simulink model "castor"  (R2021b)
settings: Solver=VariableStepAuto  StartTime=0.0  StopTime=10  MaxStep=0.01  RelTol=1e-3
settings Model: Creator=Daniel  LastModifiedBy=Daniel

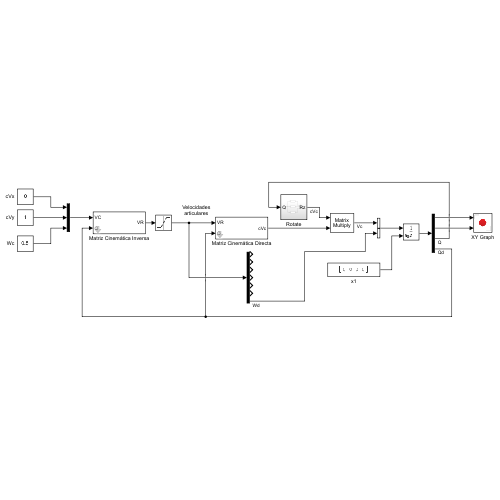
[thumbnail: Simulink's stored preview of the top-level diagram]
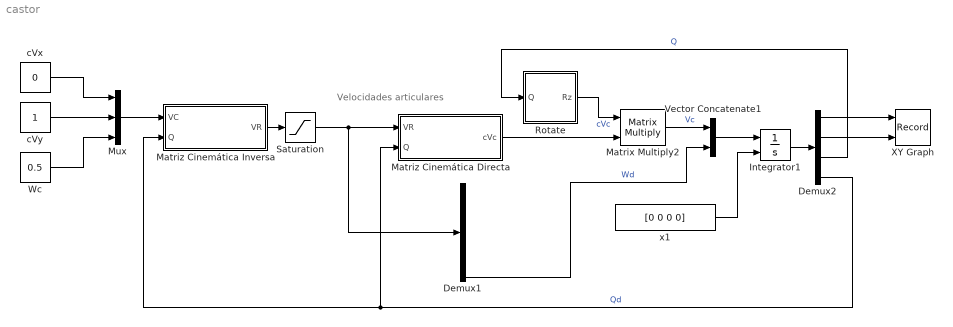
== system castor ==
  note: Velocidades
      | articulares
  Demux1 : Demux  Outputs=7
  Demux2 : Demux
  Integrator1 : Integrator  InitialConditionSource=external
  Matrix Multiply2 : Product  Multiplication=Matrix(*)
  Matriz Cinemática Directa : Subsystem  mask{d1=0.05, d2=0.05, d3=0.05, d4=0.05}
      mask prompts: d1 "Traction Wheel1 Offset"; d2 "Traction Wheel2 Offset"; d3 "Steering Offset"; d4 "Steering Length"
  Matriz Cinemática Inversa : Subsystem  mask{d1=0.05, d2=0.05, d3=0.05, d4=0.05}
      mask prompts: d1 "Traction Wheel1 Offset"; d2 "Traction Wheel2 Offset"; d3 "Steering Offset"; d4 "Steering Length"
  Mux : Mux  Inputs=3
  Rotate : Subsystem
  Saturation : Saturate  UpperLimit=1.5  LowerLimit=-1.5
  Vector Concatenate1 : Concatenate
  Wc : Constant  Value=0.5
  XY Graph : Record  FileSettingsInternal="{\"entries\":[{\"content\":{\"excelSettings\":{\"content\":{},\"type\":\"Streamout.ExcelSettings\"}},\"type\":\"Streamout.FileSettingStorage\",\"uuid\":\"8fa1ceeb-e964-410d-976c-c7ffbbaa36bc\"}],\"packageUris\":[\"http://schema.mathworks.com/mf0/streamout_blocks/R2020a\"],\"version\":\"1.0\"}"  Layout=[1 1]  SignalsInternal="{\"entries\":[{\"content\":{\"signals\":[{\"content\":{\"blockPath\":[\"castor2/XY Graph\"],\"channel\":[],\"dimensions\":[1,1],\"domain\":\"castor2/XY Graph\",\"lineColor\":\"#a2142f\",\"plots\":[1],\"port\":1,\"sid\":[],\"signalID\":9798,\"signalName\":\"Demux2:1\"},\"type\":\"RecordBlkView.Signal\",\"uuid\":\"1ec62843-dc20-4b59-a0ac-6be1d167a8ea\"},{\"content\":{\"blockPath\":[\"castor2/XY Graph\"],\"channel\":[],\"dimensions\":[1,1],\"domain\":\"castor2/XY Graph\",\"lineColor\":\"#139fff\",\"plots\":[1],\"port\":2,\"sid\":[],\"signalID\":9801,\"signalName\":\"Demux2:2\"},\"type\":\"RecordBlkView.Signal\",\"uuid\":\"d84d3f67-0fcd-4b67-8c3b-9ed586aa9fc8\"}]},\"type\":\"RecordBlkView.InputSignals\",\"uuid\":\"770f3f25-a40e-4ee6-82e0-d0dfc6b51bd0\"}],\"packageUris\":[\"http://schema.mathworks.com/mf0/streamout_blocks/R2020a\"],\"version\":\"1.0\"}"  VisualizationBindings="{\"xyplotplugin\":{\"info\":[{\"series\":[{\"bindingParametersList\":[{\"parameter\":\"X-Axis\",\"signalID\":9798,\"signalName\":\"Demux2:1\"},{\"parameter\":\"Y-Axis\",\"signalID\":9801,\"signalName\":\"Demux2:2\"}],\"seriesID\":61284}],\"subplotID\":1}]}}"  CompatibilityTag=XY
  cVx : Constant  Value=0
  cVy : Constant
  x1 : Constant  Value=[0 0 0 0]  SampleTime=-1
  wires:
  cVy/1 -> Mux/2
  cVx/1 -> Mux/1
  Demux1/7 -> Vector Concatenate1/2  "Wd"
  Matriz Cinemática Directa/1(cVc) -> Matrix Multiply2/2
  Rotate/1(Rz) -> Matrix Multiply2/1  "cVc"
  Matrix Multiply2/1 -> Vector Concatenate1/1  "Vc"
  Vector Concatenate1/1 -> Integrator1/1
  x1/1 -> Integrator1/2
  Integrator1/1 -> Demux2/1
  Demux2/1 -> XY Graph/1
  Demux2/2 -> XY Graph/2
  Mux/1 -> Matriz Cinemática Inversa/1(VC)
  Demux2/3 -> Rotate/1(Q)  "Q"
  Saturation/1 -> Demux1/1, Matriz Cinemática Directa/1(VR)
  Demux2/4 -> Matriz Cinemática Directa/2(Q), Matriz Cinemática Inversa/2(Q)  "Qd"
  Wc/1 -> Mux/3
  Matriz Cinemática Inversa/1(VR) -> Saturation/1

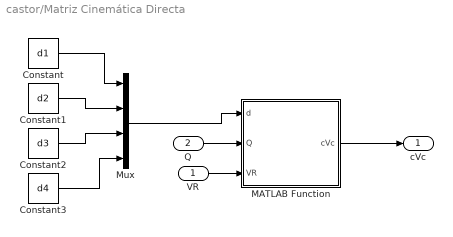
== system castor/Matriz Cinemática Directa ==
  VR : Inport
  Q : Inport  Port=2
  Constant : Constant  Value=d1
  Constant1 : Constant  Value=d2
  Constant2 : Constant  Value=d3
  Constant3 : Constant  Value=d4
  MATLAB Function : MATLAB Function  TreatAsAtomicUnit=on
  Mux : Mux
  cVc : Outport
  wires:
  VR/1 -> MATLAB Function/3(VR)
  MATLAB Function/1(cVc) -> cVc/1
  Constant1/1 -> Mux/2
  Constant2/1 -> Mux/3
  Constant/1 -> Mux/1
  Constant3/1 -> Mux/4
  Mux/1 -> MATLAB Function/1(d)
  Q/1 -> MATLAB Function/2(Q)

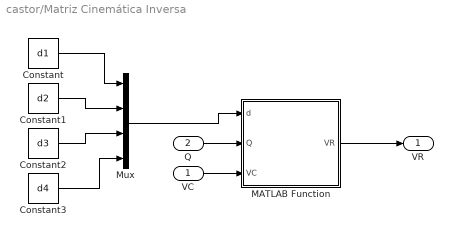
== system castor/Matriz Cinemática Inversa ==
  VC : Inport
  Q : Inport  Port=2
  Constant : Constant  Value=d1
  Constant1 : Constant  Value=d2
  Constant2 : Constant  Value=d3
  Constant3 : Constant  Value=d4
  MATLAB Function : MATLAB Function  TreatAsAtomicUnit=on
  Mux : Mux
  VR : Outport
  wires:
  Q/1 -> MATLAB Function/2(Q)
  MATLAB Function/1(VR) -> VR/1
  Constant1/1 -> Mux/2
  Constant2/1 -> Mux/3
  Constant/1 -> Mux/1
  Constant3/1 -> Mux/4
  Mux/1 -> MATLAB Function/1(d)
  VC/1 -> MATLAB Function/3(VC)

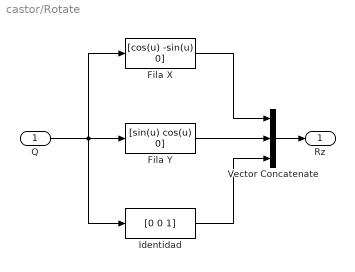
== system castor/Rotate ==
  Q : Inport
  Fila X : MATLABFcn  MATLABFcn=[cos(u) -sin(u) 0]  OutputDimensions=[1 3]  Output1D=off
  Fila Y : MATLABFcn  MATLABFcn=[sin(u) cos(u) 0]  OutputDimensions=[1 3]  Output1D=off
  Identidad : MATLABFcn  MATLABFcn=[0 0 1]  OutputDimensions=[1 3]  Output1D=off
  Vector Concatenate : Concatenate  NumInputs=3  Mode=Multidimensional array
  Rz : Outport
  wires:
  Q/1 -> Identidad/1, Fila Y/1, Fila X/1
  Vector Concatenate/1 -> Rz/1
  Fila Y/1 -> Vector Concatenate/2
  Fila X/1 -> Vector Concatenate/1
  Identidad/1 -> Vector Concatenate/3

== matlab function castor/Matriz Cinemática Directa/MATLAB Function ==
  data: d input; Q input; cVc output; VR input
function cVc = fcn(d,Q,VR)

    J1 = [0 0; 1 d(1); 0 1];
    J2 = [0 0; 1 -d(2); 0 1];
    J3 = [-sin(Q) -d(4)*cos(Q)-d(3) d(3); cos(Q) -d(4)*sin(Q) 0; 0 1 -1];
    
    A=[eye(3); eye(3); eye(3)];
    B=[J1 zeros(3,2) zeros(3,3); zeros(3,2) J2 zeros(3,3); zeros(3,2) zeros(3,2) J3];

    cVc = inv(A'*A)*A'*B*VR;

end

== matlab function castor/Matriz Cinemática Inversa/MATLAB Function ==
  data: d input; VR output; Q input; VC input
function VR = fcn(d,Q,VC)

    J1 = [0 0; 1 d(1); 0 1];
    J2 = [0 0; 1 -d(2); 0 1];
    J3 = [-sin(Q) -d(4)*cos(Q)-d(3) d(3); cos(Q) -d(4)*sin(Q) 0; 0 1 -1];
    
    % Creación de las matrices A y Jacobiana
    A=[eye(3); eye(3); eye(3)];
    B=[J1 zeros(3,2) zeros(3,3); zeros(3,2) J2 zeros(3,3); zeros(3,2) zeros(3,2) J3];

    VR = inv(B'*B)*B'*A*VC;

end
